simulink model "stage_current_controller_sim"  (R2015b)
settings: Solver=VariableStepAuto  StartTime=0.0  StopTime=0.01  RelTol=1e-3
values from neighbouring files (symbols this model uses):
  KI = KP/taum    (= 13.4208838161)    [Spindle_velocity_Controller.m]    (also in stage_current_controller.m = 3015.92894745; stage_current_controller_poleassign.m = 15079.6447372; stage_disturbance_observer.m = 615.137023081; stage_velocity_controller.m = 492.109618464)
  KP = omega0*J    (= 1.55822995618)    [Spindle_velocity_Controller.m]    (also in stage_current_controller.m = 3.76991118431; stage_current_controller_poleassign.m = 15.5822995618; stage_disturbance_observer.m = 3.73476049727; stage_postion_controller.m = 6.28318530718)
  Lq = 3*10^-3    (= 0.003)    [stage_current_controller.m]    (also in stage_current_controller_poleassign.m = 0.0031; stage_disturbance_observer.m; stage_postion_controller.m)
  R = 3    [stage_current_controller.m]    (also in stage_current_controller_poleassign.m; stage_disturbance_observer.m; stage_postion_controller.m)
  ts = 10^-3    (= 0.001)    [Spindle_velocity_Controller.m]    (also in stage_current_controller.m = 0.0001; stage_current_controller_poleassign.m = 0.000125; stage_disturbance_observer.m = 0.0005; stage_postion_controller.m = 0.0005)
libraries: cstblocks x1
settings Model: Creator=隆貴  LastModifiedBy=隆貴

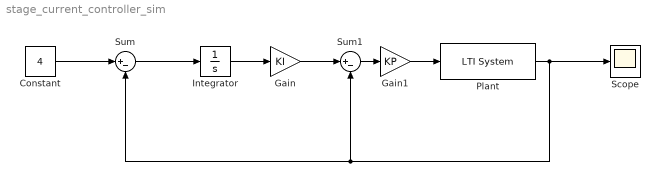
== system stage_current_controller_sim ==
  Constant : Constant  Value=4
  Gain : Gain  Gain=KI
  Gain1 : Gain  Gain=KP
  Integrator : Integrator
  Plant : cstblocks/LTI System  sys=c2d(tf(1,[Lq R]),ts)  IC=[]
  Scope : Scope
  Sum : Sum  Inputs=|+-
  Sum1 : Sum  Inputs=|+-
  wires:
  Plant/1 -> Sum/2, Sum1/2, Scope/1
  Constant/1 -> Sum/1
  Integrator/1 -> Gain/1
  Sum/1 -> Integrator/1
  Gain/1 -> Sum1/1
  Sum1/1 -> Gain1/1
  Gain1/1 -> Plant/1
